simulink library "Linkage_Arms"  (R2026a)
settings: Solver=VariableStepAuto
undefined symbols (not defined in the file): Ac, Af, Ar, bcr_mass, clr_bcr, clr_conn_la, clr_conn_pullrod, clr_conn_rod, clr_la, clr_laf, clr_lar, clr_pullrod, clr_rod, clr_ua, hp_arb, hp_bcr_pivot, hp_bcr_shock_heave, hp_bcr_shock_roll, hp_in_f_la, hp_in_f_ua, hp_in_r_la, hp_in_r_ua, hp_la_arb, hp_out_f_la, hp_out_la, hp_out_r_la, hp_out_ua, hp_pullrod_in, hp_pullrod_out, hp_pushrod_in, hp_spr_bcr, hp_spr_bot, hp_uar_rod, hp_upr_rod, la_mass, laf_mass, lar_mass, opc_bcr, opc_conn_la, opc_conn_pullrod, opc_conn_rod, opc_la, opc_laf, opc_lar, opc_pullrod, opc_rod, opc_ua, pullrod_mass, radius_bcr, radius_la, radius_laf, radius_lar, radius_pullrod, radius_rod, radius_ua, rod_mass, size_conn_la, size_conn_pullrod, size_conn_rod, ua_mass ... (+3)
libraries: Suspension_Utilities x29, sm_lib x25
(part 1 of 2)
Description:
  | Component of Simscape Vehicle Templates Library
  | 
  | Copyright 2018-2026 The MathWorks, Inc.
settings Model: Creator=smiller  LastModifiedBy=smiller

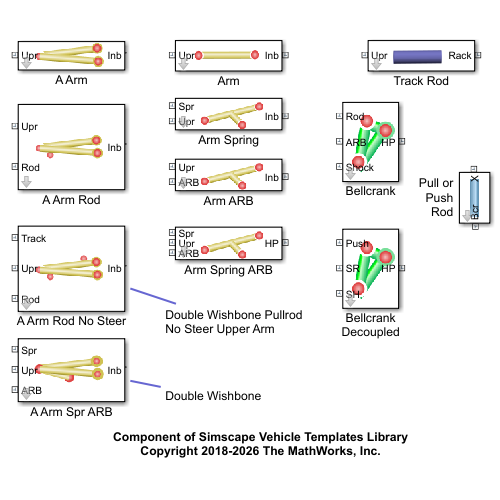
[thumbnail: Simulink's stored preview of the top-level diagram]
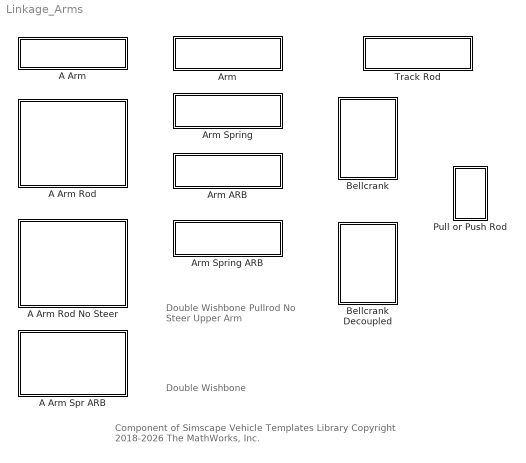
== system Linkage_Arms ==
  note: Component of Simscape Vehicle Templates Library
      | Copyright 2018-2026 The MathWorks, Inc.
  note: Double Wishbone Pullrod
      | No Steer Upper Arm
  note: Double Wishbone
  A Arm : Subsystem  mask(A-Arm){popup_leftRight=Left, hp_in_f=hp_in_f_ua, hp_in_r=hp_in_r_ua, hp_out=hp_out_ua, arm_mass=ua_mass, clr_arm=clr_ua, opc_arm=opc_ua, radius_arm=radius_ua}
      mask prompts: popup_leftRight "Left/Right"; hp_in_f "Inboard Front [xyz] (m)"; hp_in_r "Inboard Rear [xyz] (m)"; hp_out "Outboard [xyz] (m)"; arm_mass "Mass (kg)"; clr_arm "Color [RGB]"; opc_arm "Opacity (0-1)"; radius_arm "Radius (m)"
      mask help: This subsystem models a A-arm for a vehicle suspension. It can be configured to have one or two attachment points to the chassis. There are connections to the chassis and the upright.
      mask init:
      | if(popup_leftRight == 1)
      |     rhs_susp = 1;
      | elseif(popup_leftRight == 2)
      |     rhs_susp = -1;
      | end
      | 
      | rhs_hp = [1 rhs_susp 1];
      mask TypeOptions popup_leftRight: Left | Right
      mask TypeOptions clr_arm: Arm F/clr_solid | Arm R/clr_solid
      mask TypeOptions opc_arm: Arm F/opc_solid | Arm R/opc_solid
      mask TypeOptions radius_arm: Arm F/rad_solid | Arm R/rad_solid
      mask DialogControl cont_a_arm Prompt: A-Arm
      mask DialogControl cont_vis_arm Prompt: Visualization
      mask Display: image('sm_car_vehicle_linkage_dw_ua_IMAGE.png');
  A Arm Rod : Subsystem  mask(A-Arm with Rod Connection){popup_leftRight=Left, hp_in_f=hp_in_f_ua, hp_in_r=hp_in_r_ua, hp_out=hp_out_ua, hp_rod=hp_pullrod_out, arm_mass=ua_mass, clr_arm=clr_ua, opc_arm=opc_ua, radius_arm=radius_ua}
      mask prompts: popup_leftRight "Left/Right"; hp_in_f "Inboard Front [xyz] (m)"; hp_in_r "Inboard Rear [xyz] (m)"; hp_out "Outboard [xyz] (m)"; hp_rod "Rod [xyz] (m)"; arm_mass "Mass (kg)"; clr_arm "Color [RGB]"; opc_arm "Opacity (0-1)"; radius_arm "Radius (m)"
      mask help: This subsystem models a A-arm for a vehicle suspension. It can be configured to have one or two attachment points to the chassis. There are frames for connecting to the chassis, upright and a rod.
      mask init:
      | if(popup_leftRight == 1)
      |     rhs_susp = 1;
      | elseif(popup_leftRight == 2)
      |     rhs_susp = -1;
      | end
      | 
      | rhs_hp = [1 rhs_susp 1];
      mask TypeOptions popup_leftRight: Left | Right
      mask TypeOptions clr_arm: Arm F/clr_solid | Arm R/clr_solid
      mask TypeOptions opc_arm: Arm F/opc_solid | Arm R/opc_solid
      mask TypeOptions radius_arm: Arm F/rad_solid | Arm R/rad_solid
      mask DialogControl cont_a_arm Prompt: A-Arm
      mask DialogControl cont_vis_arm Prompt: Visualization
      mask Display: image('sm_car_vehicle_linkage_dw_pullrod_ua_IMAGE.png');
  A Arm Rod No Steer : Subsystem  mask(A-Arm with Rod and Track Rod Connections){popup_leftRight=Left, hp_in_f=hp_in_f_ua, hp_in_r=hp_in_r_ua, hp_r_upr=hp_uar_rod, hp_out=hp_out_ua, hp_rod=hp_pullrod_out, ua_mass=ua_mass, clr_solid=clr_ua, opc_solid=opc_ua, rad_solid=radius_ua}
      mask prompts: popup_leftRight "Left/Right"; hp_in_f "Inboard Front [xyz] (m)"; hp_in_r "Inboard Rear [xyz] (m)"; hp_r_upr "Inboard Rear to Upright [xyz] (m)"; hp_out "Outboard [xyz] (m)"; hp_rod "Rod [xyz] (m)"; ua_mass "Mass (kg)"; clr_solid "Color [RGB]"; opc_solid "Opacity (0-1)"; rad_solid "Radius (m)"
      mask help: This subsystem models a A-arm for a vehicle suspension. It can be configured to have one or two attachment points to the chassis. There are frames for connecting to the chassis, upright, rod, and track rod.
      mask init:
      | if(popup_leftRight == 1)
      |     rhs_susp = 1;
      | elseif(popup_leftRight == 2)
      |     rhs_susp = -1;
      | end
      | 
      | rhs_hp = [1 rhs_susp 1];
      mask TypeOptions popup_leftRight: Left | Right
      mask TypeOptions clr_solid: Arm F/clr_solid | Arm R/clr_solid | Arm Rod/clr_solid
      mask TypeOptions opc_solid: Arm F/opc_solid | Arm R/opc_solid | Arm Rod/opc_solid
      mask TypeOptions rad_solid: Arm F/rad_solid | Arm R/rad_solid | Arm Rod/rad_solid
      mask DialogControl cont_a_arm Prompt: A-Arm
      mask DialogControl cont_vis_ua Prompt: Visualization
      mask Display: image('sm_car_vehicle_linkage_dw_pullrod_noSteer_ua_IMAGE.png');
  A Arm Spr ARB : Subsystem  mask(A-Arm with Spring and ARB attachment){popup_leftRight=Left, hp_in_f=hp_in_f_la, hp_in_r=hp_in_r_la, hp_out=hp_out_la, hp_spr=hp_spr_bot, hp_arb=hp_la_arb, arm_mass=la_mass, clr_arm=clr_la, opc_arm=opc_la, radius_arm=radius_la}
      mask prompts: popup_leftRight "Left/Right"; hp_in_f "Inboard Front [xyz] (m)"; hp_in_r "Inboard Rear [xyz] (m)"; hp_out "Outboard [xyz] (m)"; hp_spr "Spring [xyz] (m)"; hp_arb "Anti-Roll Bar [xyz] (m)"; arm_mass "Mass (kg)"; clr_arm "Color [RGB]"; opc_arm "Opacity (0-1)"; radius_arm "Radius (m)"
      mask help: This subsystem models an arm of a wishbone suspension. It can be configured to have one or two attachment points to the chassis. There are connections to the upright, spring, and anti-roll bar.
      mask init:
      | % Set parameter for mirroring (+y or -y)
      | if(popup_leftRight == 1)
      |     rhs_susp = 1;
      | elseif(popup_leftRight == 2)
      |     rhs_susp = -1;
      | end
      | 
      | rhs_hp = [1 rhs_susp 1];
      mask Help: web ('sm_car_lower_arm_help.html')
      mask TypeOptions popup_leftRight: Left | Right
      mask TypeOptions clr_arm: Arm ARB/clr_solid | Arm F/clr_solid | Arm R/clr_solid | Arm Spring/clr_solid
      mask TypeOptions opc_arm: Arm ARB/opc_solid | Arm F/opc_solid | Arm R/opc_solid | Arm Spring/opc_solid
      mask TypeOptions radius_arm: Arm ARB/rad_solid | Arm F/rad_solid | Arm R/rad_solid | Arm Spring/rad_solid
      mask DialogControl cont_a_arm Prompt: A-Arm
      mask DialogControl cont_vis_arm Prompt: Visualization
      mask Display: image('sm_car_vehicle_linkage_dw_la_IMAGE.png');
  Arm : Subsystem  VariantControl=Steer  mask(Arm){popup_leftRight=Left, hp_in=hp_in_r_la, hp_out=hp_out_r_la, rod_mass=lar_mass, clr_conn_rod=clr_conn_la, opc_conn_rod=opc_conn_la, size_conn_rod=size_conn_la, clr_rod=clr_lar, opc_rod=opc_lar, radius_rod=radius_lar}
      mask prompts: popup_leftRight "Left/Right"; hp_in "Inboard [xyz] (m)"; hp_out "Outboard [xyz] (m)"; rod_mass "Mass (kg)"
      mask help: Rigid arm with two connection points.
      mask init:
      | if(popup_leftRight == 1)
      |     rhs_rod = 1;
      | elseif(popup_leftRight == 2)
      |     rhs_rod = -1;
      | end
      mask TypeOptions popup_leftRight: Left | Right
      mask TypeOptions rod_mass: Arm/Mass
      mask TypeOptions clr_conn_rod:
      | Vis
      | HP
      | Upr/GraphicDiffuseColor | Vis
      | HP
      | Inb/GraphicDiffuseColor
      mask TypeOptions opc_conn_rod:
      | Vis
      | HP
      | Upr/GraphicOpacity | Vis
      | HP
      | Inb/GraphicOpacity
      mask TypeOptions clr_rod: Arm/clr_solid
      mask TypeOptions opc_rod: Arm/opc_solid
      mask TypeOptions radius_rod: Arm/rad_solid
      mask DialogControl cont_rod Prompt: Rod
      mask DialogControl grp_rod Prompt: Rod
      mask DialogControl cont_vis_rod Prompt: Visualization
      mask DialogControl text_clr_rod Prompt: Color [RGB]
      mask DialogControl text_opc_rod Prompt: Opacity (0-1)
      mask DialogControl text_size_rod Prompt: Radius (m)
      mask DialogControl text_conn_rod Prompt: Connections
      mask DialogControl text_rod_rod Prompt: Rod
      mask Display: image('sm_car_vehicle_linkage_link_IMAGE.png');
  Arm ARB : Subsystem  VariantControl=Steer  mask(Arm with Anti-Roll Bar Connection){popup_leftRight=Left, hp_in=hp_in_r_la, hp_out=hp_out_r_la, hp_arb=hp_arb, rod_mass=lar_mass, clr_conn_rod=clr_conn_la, opc_conn_rod=opc_conn_la, size_conn_rod=size_conn_la, clr_rod=clr_laf, opc_rod=opc_laf, radius_rod=radius_laf}
      mask prompts: popup_leftRight "Left/Right"; hp_in "Inboard [xyz] (m)"; hp_out "Outboard [xyz] (m)"; hp_arb "ARB Mount [xyz] (m)"; rod_mass "Mass (kg)"
      mask help: Rigid arm with two ends and a frame for connecting to the anti-roll bar.
      mask init:
      | if(popup_leftRight == 1)
      |     rhs_rod = 1;
      | elseif(popup_leftRight == 2)
      |     rhs_rod = -1;
      | end
      mask TypeOptions popup_leftRight: Left | Right
      mask TypeOptions rod_mass: Arm/Mass
      mask TypeOptions clr_conn_rod:
      | Vis
      | HP
      | Upright/GraphicDiffuseColor | Vis
      | HP
      | Inb/GraphicDiffuseColor
      mask TypeOptions opc_conn_rod:
      | Vis
      | HP
      | Upright/GraphicOpacity | Vis
      | HP
      | Inb/GraphicOpacity
      mask TypeOptions clr_rod: Arm/clr_solid
      mask TypeOptions opc_rod: Arm/opc_solid
      mask TypeOptions radius_rod: Arm/rad_solid
      mask DialogControl cont_rod Prompt: Rod
      mask DialogControl grp_rod Prompt: Rod
      mask DialogControl cont_vis_rod Prompt: Visualization
      mask DialogControl text_clr_rod Prompt: Color [RGB]
      mask DialogControl text_opc_rod Prompt: Opacity (0-1)
      mask DialogControl text_size_rod Prompt: Radius (m)
      mask DialogControl text_conn_rod Prompt: Connections
      mask DialogControl text_rod_rod Prompt: Rod
      mask Display: image('sm_car_vehicle_linkage_link_s2f_IMAGE.png');
  Arm Spring : Subsystem  VariantControl=Steer  mask(Arm with Spring Connection){popup_leftRight=Left, hp_in=hp_in_f_la, hp_out=hp_out_f_la, hp_spr=hp_spr_bot, rod_mass=laf_mass, clr_conn_rod=clr_conn_la, opc_conn_rod=opc_conn_la, size_conn_rod=size_conn_la, clr_rod=clr_laf, opc_rod=opc_laf, radius_rod=radius_laf}
      mask prompts: popup_leftRight "Left/Right"; hp_in "Inboard [xyz] (m)"; hp_out "Outboard [xyz] (m)"; hp_spr "Spring Mount [xyz] (m)"; rod_mass "Mass (kg)"
      mask help: Rigid arm with two ends and a frame for connecting to the spring.
      mask init:
      | if(popup_leftRight == 1)
      |     rhs_rod = 1;
      | elseif(popup_leftRight == 2)
      |     rhs_rod = -1;
      | end
      mask TypeOptions popup_leftRight: Left | Right
      mask TypeOptions rod_mass: Arm/Mass
      mask TypeOptions clr_conn_rod:
      | Vis
      | HP
      | Upr/GraphicDiffuseColor | Vis
      | HP
      | Inb/GraphicDiffuseColor
      mask TypeOptions opc_conn_rod:
      | Vis
      | HP
      | Upr/GraphicOpacity | Vis
      | HP
      | Inb/GraphicOpacity
      mask TypeOptions clr_rod: Arm/clr_solid
      mask TypeOptions opc_rod: Arm/opc_solid
      mask TypeOptions radius_rod: Arm/rad_solid
      mask DialogControl cont_rod Prompt: Rod
      mask DialogControl grp_rod Prompt: Rod
      mask DialogControl cont_vis_rod Prompt: Visualization
      mask DialogControl text_clr_rod Prompt: Color [RGB]
      mask DialogControl text_opc_rod Prompt: Opacity (0-1)
      mask DialogControl text_size_rod Prompt: Radius (m)
      mask DialogControl text_conn_rod Prompt: Connections
      mask DialogControl text_rod_rod Prompt: Rod
      mask Display: image('sm_car_vehicle_linkage_link_s2f_IMAGE.png');
  Arm Spring ARB : Subsystem  VariantControl=Steer  mask(Arm with Connections to Spring and Anti-Roll Bar){popup_leftRight=Left, hp_in=hp_in_r_la, hp_out=hp_out_r_la, hp_spr=hp_spr_bot, hp_arb=hp_arb, rod_mass=laf_mass, clr_conn_rod=clr_conn_la, opc_conn_rod=opc_conn_la, size_conn_rod=size_conn_la, clr_rod=clr_laf, opc_rod=opc_laf, radius_rod=radius_laf}
      mask prompts: popup_leftRight "Left/Right"; hp_in "Inboard [xyz] (m)"; hp_out "Outboard [xyz] (m)"; hp_spr "Spring Mount [xyz] (m)"; hp_arb "ARB Mount [xyz] (m)"; rod_mass "Mass (kg)"
      mask help: Rigid arm with two ends and frames for connecting to the spring and anti-roll bar.
      mask init:
      | if(popup_leftRight == 1)
      |     rhs_rod = 1;
      | elseif(popup_leftRight == 2)
      |     rhs_rod = -1;
      | end
      mask TypeOptions popup_leftRight: Left | Right
      mask TypeOptions rod_mass: Arm/Mass
      mask TypeOptions clr_conn_rod:
      | Vis
      | Upright
      | Steer/GraphicDiffuseColor | Vis
      | Rack
      | Rod/GraphicDiffuseColor
      mask TypeOptions opc_conn_rod:
      | Vis
      | Upright
      | Steer/GraphicOpacity | Vis
      | Rack
      | Rod/GraphicOpacity
      mask TypeOptions clr_rod: Arm/clr_solid
      mask TypeOptions opc_rod: Arm/opc_solid
      mask TypeOptions radius_rod: Arm/rad_solid
      mask DialogControl cont_rod Prompt: Rod
      mask DialogControl grp_rod Prompt: Rod
      mask DialogControl cont_vis_rod Prompt: Visualization
      mask DialogControl text_clr_rod Prompt: Color [RGB]
      mask DialogControl text_opc_rod Prompt: Opacity (0-1)
      mask DialogControl text_size_rod Prompt: Radius (m)
      mask DialogControl text_conn_rod Prompt: Connections
      mask DialogControl text_rod_rod Prompt: Rod
      mask Display: image('sm_car_vehicle_linkage_link_s2f_IMAGE.png');
  Bellcrank : Subsystem  mask(Bellcrank){popup_leftRight=Left, hp_bcr_pivot=hp_bcr_pivot, hp_bcr_shock=hp_spr_bcr, hp_rod=hp_pullrod_in, hp_arb=hp_arb, bcr_mass=bcr_mass, clr_bcr=clr_bcr, opc_bcr=opc_bcr, radius_bcr=radius_bcr}
      mask prompts: popup_leftRight "Left/Right"; hp_bcr_pivot "HP Bellcrank Pivot [xyz] (m)"; hp_bcr_shock "HP Bellcrank Shock [xyz] (m)"; hp_rod "HP Bellcrank Rod [xyz] (m)"; hp_arb "HP Bellcrank ARB [xyz] (m)"; bcr_mass "Mass (kg)"; clr_bcr "Color [RGB]"; opc_bcr "Opacity (0-1)"; radius_bcr "Radius (m)"
      mask help: Models a bellcrank with one pivot and 3 attachment points. The axis of the pivot is normal to the plane formed by the pivot, connection to the rod, and connection to the shock.
      mask init:
      | if(popup_leftRight == 1)
      |     rhs_susp = 1;
      | elseif(popup_leftRight == 2)
      |     rhs_susp = -1;
      | end
      | 
      | rhs_hp = [1 rhs_susp 1];
      mask TypeOptions popup_leftRight: Left | Right
      mask TypeOptions clr_bcr: Arm Pivot ARB/clr_solid | Arm Pivot Rod/clr_solid | Arm Pivot Shock/clr_solid | Arm Rod Shock/clr_solid
      mask TypeOptions opc_bcr: Arm Pivot ARB/opc_solid | Arm Pivot Rod/opc_solid | Arm Pivot Shock/opc_solid | Arm Rod Shock/opc_solid
      mask TypeOptions radius_bcr: Arm Pivot ARB/rad_solid | Arm Pivot Rod/rad_solid | Arm Pivot Shock/rad_solid | Arm Rod Shock/rad_solid
      mask DialogControl cont_ua Prompt: UA
      mask DialogControl cont_vis_ua Prompt: Visualization
      mask Display: image('sm_car_vehicle_linkage_bellcrank_IMAGE.png');
  Bellcrank Decoupled : Subsystem  mask(Bellcrank){popup_leftRight=Left, hp_bcr_pivot=hp_bcr_pivot, hp_bcr_shock_heave=hp_bcr_shock_heave, hp_bcr_shock_roll=hp_bcr_shock_roll, hp_pushrod=hp_pushrod_in, bcr_mass=bcr_mass, clr_bcr=clr_bcr, opc_bcr=opc_bcr, radius_bcr=radius_bcr}
      mask prompts: popup_leftRight "Left/Right"; hp_bcr_pivot "HP Bellcrank Pivot [xyz] (m)"; hp_bcr_shock_heave "HP Bellcrank Shock Heave [xyz] (m)"; hp_bcr_shock_roll "HP Bellcrank Shock Roll [xyz] (m)"; hp_pushrod "HP Bellcrank Pushrod [xyz] (m)"; bcr_mass "Mass (kg)"; clr_bcr "Color [RGB]"; opc_bcr "Opacity (0-1)"; radius_bcr "Radius (m)"
      mask help: Models a bellcrank with one pivot and 3 attachment points. The axis of the pivot is normal to the plane formed by the pivot, connection to the pushrod, and connection to the shock.
      mask init:
      | if(popup_leftRight == 1)
      |     rhs_susp = 1;
      |     %hp_shock_roll = hp_bcr_shock_roll; % Use left value
      | elseif(popup_leftRight == 2)
      |     rhs_susp = -1;
      |     % Code to mirror hardpoint about vehicle xz plane 
      |     % and the plane defined by the bellcrank pivot axis
      |     % and the y axis of the vehicle
      |     % Code not used so that points can be specified independently
      |     % Left here as a reference.
      |     %{
      |     a1 = atan2(hp_pushrod(1)-hp_bcr_pivot(1)   ,hp_pushrod(3)-hp_bcr_pivot(3));
      |     a2 = atan2(hp_bcr_shock_roll(1)-hp_bcr_pivot(1),hp_bcr_shock_roll(3)-hp_bcr_pivot(3));
      |     d_roll2piv = norm(hp_bcr_shock_roll([1 3])-hp_bcr_pivot([1 3]));
      |     d_roll_mirror_axis = d_roll2piv*cos(a2-a1);
      |     mirr_dx = d_roll_mirror_axis*sin(a1);
      |     mirr_dz = d_roll_mirror_axis*cos(a1);
      |     hp_shock_roll = ...
      |         [hp_bcr_shock_roll(1)-2*mirr_dx -hp_bcr_shock_roll(2) hp_bcr_shock_roll(3)-2*mirr_dz];
      |     %}
      | end
      | 
      | rhs_hp = [1 rhs_susp 1];
      mask TypeOptions popup_leftRight: Left | Right
      mask TypeOptions clr_bcr: Arm Pivot Shock Roll/clr_solid | Arm Pivot Push/clr_solid | Arm Pivot Shock Heave/clr_solid | Arm Push Shock/clr_solid
      mask TypeOptions opc_bcr: Arm Pivot Shock Roll/opc_solid | Arm Pivot Push/opc_solid | Arm Pivot Shock Heave/opc_solid | Arm Push Shock/opc_solid
      mask TypeOptions radius_bcr: Arm Pivot Shock Roll/rad_solid | Arm Pivot Push/rad_solid | Arm Pivot Shock Heave/rad_solid | Arm Push Shock/rad_solid
      mask DialogControl cont_ua Prompt: UA
      mask DialogControl cont_vis_ua Prompt: Visualization
      mask Display: image('sm_car_vehicle_linkage_bellcrank_IMAGE.png');
  Pull or Push Rod : Subsystem  VariantControl=Steer  mask(Rod){popup_leftRight=Left, hp_in=hp_pullrod_in, hp_out=hp_pullrod_out, rod_mass=pullrod_mass, clr_conn_rod=clr_conn_pullrod, opc_conn_rod=opc_conn_pullrod, size_conn_rod=size_conn_pullrod, clr_rod=clr_pullrod, opc_rod=opc_pullrod, radius_rod=radius_pullrod}
      mask prompts: popup_leftRight "Left/Right"; hp_in "Bellcrank [xyz] (m)"; hp_out "Arm / Upright [xyz] (m)"; rod_mass "Mass (kg)"
      mask help: Rod connecting two hard points
      mask init:
      | if(popup_leftRight == 1)
      |     rhs_rod = 1;
      | elseif(popup_leftRight == 2)
      |     rhs_rod = -1;
      | end
      mask TypeOptions popup_leftRight: Left | Right
      mask TypeOptions rod_mass: Rod/Mass
      mask TypeOptions clr_conn_rod:
      | Vis
      | Pushrod
      | X/GraphicDiffuseColor | Vis
      | Pushrod
      | Crank/GraphicDiffuseColor
      mask TypeOptions opc_conn_rod:
      | Vis
      | Pushrod
      | X/GraphicOpacity | Vis
      | Pushrod
      | Crank/GraphicOpacity
      mask TypeOptions clr_rod: Rod/clr_solid
      mask TypeOptions opc_rod: Rod/opc_solid
      mask TypeOptions radius_rod: Rod/rad_solid
      mask DialogControl cont_rod Prompt: Rod
      mask DialogControl grp_rod Prompt: Rod
      mask DialogControl cont_vis_rod Prompt: Visualization
      mask DialogControl text_clr_rod Prompt: Color [RGB]
      mask DialogControl text_opc_rod Prompt: Opac. (0-1)
      mask DialogControl text_size_rod Prompt: Size (m)
      mask DialogControl text_conn_rod Prompt: Connections
      mask DialogControl text_rod_rod Prompt: Rod
      mask Display: image('sm_car_vehicle_linkage_pushrod_IMAGE.png');
  Track Rod : Subsystem  VariantControl=Steer  mask(Rod){popup_leftRight=Left, hp_in=hp_uar_rod, hp_out=hp_upr_rod, rod_mass=rod_mass, clr_conn_rod=clr_conn_rod, opc_conn_rod=opc_conn_rod, size_conn_rod=size_conn_rod, clr_rod=clr_rod, opc_rod=opc_rod, radius_rod=radius_rod}
      mask prompts: popup_leftRight "Left/Right"; hp_in "Inboard [xyz] (m)"; hp_out "Outboard [xyz] (m)"; rod_mass "Mass (kg)"
      mask help: Rod connecting two hard points
      mask init:
      | if(popup_leftRight == 1)
      |     rhs_rod = 1;
      | elseif(popup_leftRight == 2)
      |     rhs_rod = -1;
      | end
      mask TypeOptions popup_leftRight: Left | Right
      mask TypeOptions rod_mass: Rod/Mass
      mask TypeOptions clr_conn_rod:
      | Vis
      | Upright
      | Steer/GraphicDiffuseColor | Vis
      | Rack
      | Rod/GraphicDiffuseColor
      mask TypeOptions opc_conn_rod:
      | Vis
      | Upright
      | Steer/GraphicOpacity | Vis
      | Rack
      | Rod/GraphicOpacity
      mask TypeOptions clr_rod: Rod/clr_solid
      mask TypeOptions opc_rod: Rod/opc_solid
      mask TypeOptions radius_rod: Rod/rad_solid
      mask DialogControl cont_rod Prompt: Rod
      mask DialogControl grp_rod Prompt: Rod
      mask DialogControl cont_vis_rod Prompt: Visualization
      mask DialogControl text_clr_rod Prompt: Color [RGB]
      mask DialogControl text_opc_rod Prompt: Opac. (0-1)
      mask DialogControl text_size_rod Prompt: Size (m)
      mask DialogControl text_conn_rod Prompt: Connections
      mask DialogControl text_rod_rod Prompt: Rod
      mask Display: image('sm_car_linkage_trackrod_IMAGE.png');

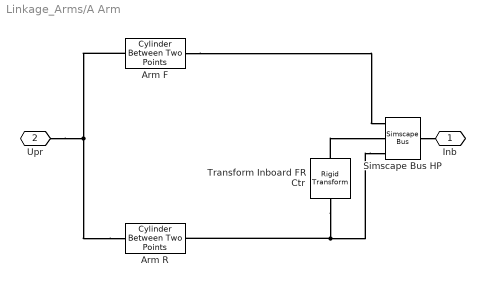
== system Linkage_Arms/A Arm ==
  Arm F : Suspension_Utilities/Cylinder Between Two Points  hp_b=hp_in_f.*rhs_hp  hp_f=hp_out.*rhs_hp  Mass=arm_mass/2  clr_solid=clr_arm  opc_solid=opc_arm  rad_solid=radius_arm
  Arm R : Suspension_Utilities/Cylinder Between Two Points  hp_b=hp_in_r.*rhs_hp  hp_f=hp_out.*rhs_hp  Mass=arm_mass/2  clr_solid=clr_arm  opc_solid=opc_arm  rad_solid=radius_arm
  Simscape Bus HP : SimscapeBus  HierarchyStrings=Af;Ac;Ar
  Transform Inboard FR Ctr : sm_lib/Frames and Transforms/Rigid Transform  RotationMethod=None  FollAlignAxisA=+X  BaseAlignAxisA=+Y  FollAlignAxisB=+Y  BaseAlignAxisB=+Z  RotationStandardAxis=+Z  RotationAngle=0.0  RotationAngleUnits=deg  RotationArbitraryAxis=[0 0 1]  RotationSequenceAxes=FollowerAxes  RotationSequence=XYX  RotationSequenceAngles=[0 0 0]  RotationSequenceAnglesUnits=deg  RotationMatrix=[1 0 0; 0 1 0; 0 0 1]  Quaternion=[1 0 0 0]  TranslationMethod=Cartesian  TranslationCartesianOffset=(hp_in_f - hp_in_r).*rhs_hp/2  TranslationCartesianOffsetUnits=m  TranslationStandardAxis=+Z  TranslationStandardOffset=0  TranslationStandardOffsetUnits=m  TranslationROffset=0  TranslationROffsetUnits=m  TranslationThetaOffset=0  TranslationThetaOffsetUnits=deg  TranslationZOffset=0  TranslationZOffsetUnits=m
  Inb : PMIOPort  Side=Right
  Upr : PMIOPort  Port=2  Side=Left
  connections:
  Arm R/RConn1 -- Upr/RConn1 -- Arm F/RConn1
  Simscape Bus HP/LConn3 -- Arm R/LConn1 -- Transform Inboard FR Ctr/LConn1
  Arm F/LConn1 -- Simscape Bus HP/LConn1
  Transform Inboard FR Ctr/RConn1 -- Simscape Bus HP/LConn2
  Simscape Bus HP/RConn1 -- Inb/RConn1

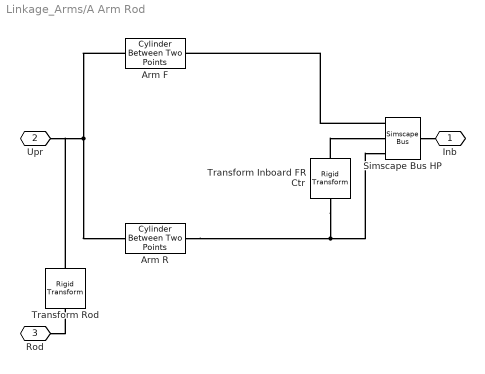
== system Linkage_Arms/A Arm Rod ==
  Arm F : Suspension_Utilities/Cylinder Between Two Points  hp_b=hp_in_f.*rhs_hp  hp_f=hp_out.*rhs_hp  Mass=ua_mass/2  clr_solid=clr_arm  opc_solid=opc_arm  rad_solid=radius_arm
  Arm R : Suspension_Utilities/Cylinder Between Two Points  hp_b=hp_in_r.*rhs_hp  hp_f=hp_out.*rhs_hp  Mass=ua_mass/2  clr_solid=clr_arm  opc_solid=opc_arm  rad_solid=radius_arm
  Simscape Bus HP : SimscapeBus  HierarchyStrings=Af;Ac;Ar
  Transform Inboard FR Ctr : sm_lib/Frames and Transforms/Rigid Transform  RotationMethod=None  FollAlignAxisA=+X  BaseAlignAxisA=+Y  FollAlignAxisB=+Y  BaseAlignAxisB=+Z  RotationStandardAxis=+Z  RotationAngle=0.0  RotationAngleUnits=deg  RotationArbitraryAxis=[0 0 1]  RotationSequenceAxes=FollowerAxes  RotationSequence=XYX  RotationSequenceAngles=[0 0 0]  RotationSequenceAnglesUnits=deg  RotationMatrix=[1 0 0; 0 1 0; 0 0 1]  Quaternion=[1 0 0 0]  TranslationMethod=Cartesian  TranslationCartesianOffset=(hp_in_f - hp_in_r).*rhs_hp/2  TranslationCartesianOffsetUnits=m  TranslationStandardAxis=+Z  TranslationStandardOffset=0  TranslationStandardOffsetUnits=m  TranslationROffset=0  TranslationROffsetUnits=m  TranslationThetaOffset=0  TranslationThetaOffsetUnits=deg  TranslationZOffset=0  TranslationZOffsetUnits=m
  Transform Rod : sm_lib/Frames and Transforms/Rigid Transform  RotationMethod=None  FollAlignAxisA=+X  BaseAlignAxisA=+Y  FollAlignAxisB=+Y  BaseAlignAxisB=+Z  RotationStandardAxis=+Z  RotationAngle=0.0  RotationAngleUnits=deg  RotationArbitraryAxis=[0 0 1]  RotationSequenceAxes=FollowerAxes  RotationSequence=XYX  RotationSequenceAngles=[0 0 0]  RotationSequenceAnglesUnits=deg  RotationMatrix=[1 0 0; 0 1 0; 0 0 1]  Quaternion=[1 0 0 0]  TranslationMethod=Cartesian  TranslationCartesianOffset=(hp_rod-hp_out).*rhs_hp  TranslationCartesianOffsetUnits=m  TranslationStandardAxis=+Z  TranslationStandardOffset=0  TranslationStandardOffsetUnits=m  TranslationROffset=0  TranslationROffsetUnits=m  TranslationThetaOffset=0  TranslationThetaOffsetUnits=deg  TranslationZOffset=0  TranslationZOffsetUnits=m
  Inb : PMIOPort  Side=Right
  Upr : PMIOPort  Port=2  Side=Left
  Rod : PMIOPort  Port=3  Side=Left
  connections:
  Rod/RConn1 -- Transform Rod/RConn1
  Simscape Bus HP/RConn1 -- Inb/RConn1
  Transform Inboard FR Ctr/RConn1 -- Simscape Bus HP/LConn2
  Transform Inboard FR Ctr/LConn1 -- Simscape Bus HP/LConn3 -- Arm R/LConn1
  Simscape Bus HP/LConn1 -- Arm F/LConn1
  Arm F/RConn1 -- Upr/RConn1 -- Transform Rod/LConn1 -- Arm R/RConn1

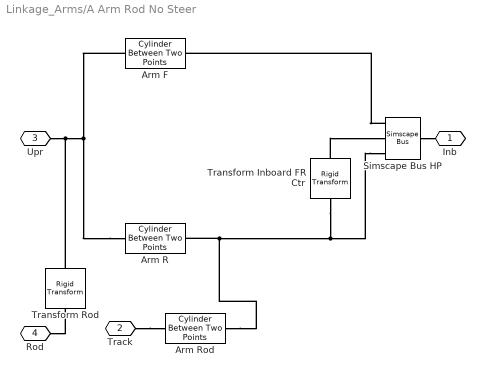
== system Linkage_Arms/A Arm Rod No Steer ==
  Arm F : Suspension_Utilities/Cylinder Between Two Points  hp_b=hp_in_f.*rhs_hp  hp_f=hp_out.*rhs_hp  Mass=ua_mass/2  clr_solid=clr_solid  opc_solid=opc_solid  rad_solid=rad_solid
  Arm R : Suspension_Utilities/Cylinder Between Two Points  hp_b=hp_in_r.*rhs_hp  hp_f=hp_out.*rhs_hp  Mass=ua_mass/2  clr_solid=clr_solid  opc_solid=opc_solid  rad_solid=rad_solid
  Arm Rod : Suspension_Utilities/Cylinder Between Two Points  hp_b=hp_in_r.*rhs_hp  hp_f=hp_r_upr.*rhs_hp  Mass=0  clr_solid=clr_solid  opc_solid=opc_solid  rad_solid=rad_solid
  Simscape Bus HP : SimscapeBus  HierarchyStrings=Af;Ac;Ar
  Transform Inboard FR Ctr : sm_lib/Frames and Transforms/Rigid Transform  RotationMethod=None  FollAlignAxisA=+X  BaseAlignAxisA=+Y  FollAlignAxisB=+Y  BaseAlignAxisB=+Z  RotationStandardAxis=+Z  RotationAngle=0.0  RotationAngleUnits=deg  RotationArbitraryAxis=[0 0 1]  RotationSequenceAxes=FollowerAxes  RotationSequence=XYX  RotationSequenceAngles=[0 0 0]  RotationSequenceAnglesUnits=deg  RotationMatrix=[1 0 0; 0 1 0; 0 0 1]  Quaternion=[1 0 0 0]  TranslationMethod=Cartesian  TranslationCartesianOffset=(hp_in_f - hp_in_r).*rhs_hp/2  TranslationCartesianOffsetUnits=m  TranslationStandardAxis=+Z  TranslationStandardOffset=0  TranslationStandardOffsetUnits=m  TranslationROffset=0  TranslationROffsetUnits=m  TranslationThetaOffset=0  TranslationThetaOffsetUnits=deg  TranslationZOffset=0  TranslationZOffsetUnits=m
  Transform Rod : sm_lib/Frames and Transforms/Rigid Transform  RotationMethod=None  FollAlignAxisA=+X  BaseAlignAxisA=+Y  FollAlignAxisB=+Y  BaseAlignAxisB=+Z  RotationStandardAxis=+Z  RotationAngle=0.0  RotationAngleUnits=deg  RotationArbitraryAxis=[0 0 1]  RotationSequenceAxes=FollowerAxes  RotationSequence=XYX  RotationSequenceAngles=[0 0 0]  RotationSequenceAnglesUnits=deg  RotationMatrix=[1 0 0; 0 1 0; 0 0 1]  Quaternion=[1 0 0 0]  TranslationMethod=Cartesian  TranslationCartesianOffset=(hp_rod-hp_out).*rhs_hp  TranslationCartesianOffsetUnits=m  TranslationStandardAxis=+Z  TranslationStandardOffset=0  TranslationStandardOffsetUnits=m  TranslationROffset=0  TranslationROffsetUnits=m  TranslationThetaOffset=0  TranslationThetaOffsetUnits=deg  TranslationZOffset=0  TranslationZOffsetUnits=m
  Inb : PMIOPort  Side=Right
  Track : PMIOPort  Port=2  Side=Left
  Upr : PMIOPort  Port=3  Side=Left
  Rod : PMIOPort  Port=4  Side=Left
  connections:
  Track/RConn1 -- Arm Rod/RConn1
  Arm R/RConn1 -- Transform Rod/LConn1 -- Upr/RConn1 -- Arm F/RConn1
  Simscape Bus HP/LConn1 -- Arm F/LConn1
  Simscape Bus HP/LConn3 -- Transform Inboard FR Ctr/LConn1 -- Arm R/LConn1 -- Arm Rod/LConn1
  Transform Inboard FR Ctr/RConn1 -- Simscape Bus HP/LConn2
  Simscape Bus HP/RConn1 -- Inb/RConn1
  Rod/RConn1 -- Transform Rod/RConn1

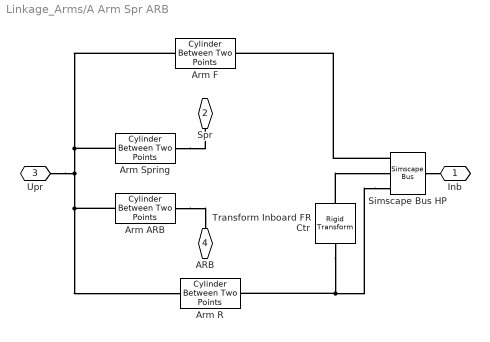
== system Linkage_Arms/A Arm Spr ARB ==
  Arm ARB : Suspension_Utilities/Cylinder Between Two Points  hp_b=hp_arb.*rhs_hp  hp_f=hp_out.*rhs_hp  Mass=0  clr_solid=clr_arm  opc_solid=opc_arm  rad_solid=radius_arm
  Arm F : Suspension_Utilities/Cylinder Between Two Points  hp_b=hp_in_f.*rhs_hp  hp_f=hp_out.*rhs_hp  Mass=arm_mass/2  clr_solid=clr_arm  opc_solid=opc_arm  rad_solid=radius_arm
  Arm R : Suspension_Utilities/Cylinder Between Two Points  hp_b=hp_in_r.*rhs_hp  hp_f=hp_out.*rhs_hp  Mass=arm_mass/2  clr_solid=clr_arm  opc_solid=opc_arm  rad_solid=radius_arm
  Arm Spring : Suspension_Utilities/Cylinder Between Two Points  hp_b=hp_spr.*rhs_hp  hp_f=hp_out.*rhs_hp  Mass=0  clr_solid=clr_arm  opc_solid=opc_arm  rad_solid=radius_arm
  Simscape Bus HP : SimscapeBus  HierarchyStrings=Af;Ac;Ar
  Transform Inboard FR Ctr : sm_lib/Frames and Transforms/Rigid Transform  RotationMethod=None  FollAlignAxisA=+X  BaseAlignAxisA=+Y  FollAlignAxisB=+Y  BaseAlignAxisB=+Z  RotationStandardAxis=+Z  RotationAngle=0.0  RotationAngleUnits=deg  RotationArbitraryAxis=[0 0 1]  RotationSequenceAxes=FollowerAxes  RotationSequence=XYX  RotationSequenceAngles=[0 0 0]  RotationSequenceAnglesUnits=deg  RotationMatrix=[1 0 0; 0 1 0; 0 0 1]  Quaternion=[1 0 0 0]  TranslationMethod=Cartesian  TranslationCartesianOffset=(hp_in_f - hp_in_r).*rhs_hp/2  TranslationCartesianOffsetUnits=m  TranslationStandardAxis=+Z  TranslationStandardOffset=0  TranslationStandardOffsetUnits=m  TranslationROffset=0  TranslationROffsetUnits=m  TranslationThetaOffset=0  TranslationThetaOffsetUnits=deg  TranslationZOffset=0  TranslationZOffsetUnits=m
  Inb : PMIOPort  Side=Right
  Spr : PMIOPort  Port=2  Side=Left
  Upr : PMIOPort  Port=3  Side=Left
  ARB : PMIOPort  Port=4  Side=Left
  connections:
  Transform Inboard FR Ctr/RConn1 -- Simscape Bus HP/LConn2
  Simscape Bus HP/RConn1 -- Inb/RConn1
  Arm Spring/LConn1 -- Spr/RConn1
  Arm F/RConn1 -- Arm R/RConn1 -- Arm ARB/RConn1 -- Upr/RConn1 -- Arm Spring/RConn1
  Simscape Bus HP/LConn3 -- Transform Inboard FR Ctr/LConn1 -- Arm R/LConn1
  Simscape Bus HP/LConn1 -- Arm F/LConn1
  Arm ARB/LConn1 -- ARB/RConn1

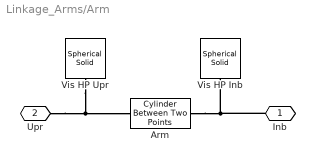
== system Linkage_Arms/Arm ==
  Arm : Suspension_Utilities/Cylinder Between Two Points  hp_b=hp_in.*[1 rhs_rod 1]  hp_f=hp_out.*[1 rhs_rod 1]  Mass=rod_mass  clr_solid=clr_rod  opc_solid=opc_rod  rad_solid=radius_rod
  Vis HP Inb : sm_lib/Body Elements/Spherical Solid  SphereRadius=size_conn_rod  SphereRadiusUnits=m  ExportEntireGeometry=off  InertiaType=CalculateFromGeometry  BasedOnType=Density  Density=0  DensityUnits=kg/m^3  Mass=1  MassUnits=kg  CenterOfMass=[0 0 0]  CenterOfMassUnits=m  MomentsOfInertia=[1 1 1]  MomentsOfInertiaUnits=kg*m^2  ProductsOfInertia=[0 0 0]  ProductsOfInertiaUnits=kg*m^2  GraphicType=FromGeometry  MarkerShape=Sphere  MarkerSize=10  GraphicVisPropType=SimpleVisualProperties  GraphicDiffuseColor=clr_conn_rod  GraphicOpacity=opc_conn_rod  GraphicSpecularColor=[0.5 0.5 0.5 1.0]  GraphicAmbientColor=[0.15 0.15 0.15 1.0]  GraphicEmissiveColor=[0.0 0.0 0.0 1.0]  GraphicShininess=75  DoExposeReferenceFrame=on  SerializedFrames=<Frames/>
  Vis HP Upr : sm_lib/Body Elements/Spherical Solid  SphereRadius=size_conn_rod  SphereRadiusUnits=m  ExportEntireGeometry=off  InertiaType=CalculateFromGeometry  BasedOnType=Density  Density=0  DensityUnits=kg/m^3  Mass=1  MassUnits=kg  CenterOfMass=[0 0 0]  CenterOfMassUnits=m  MomentsOfInertia=[1 1 1]  MomentsOfInertiaUnits=kg*m^2  ProductsOfInertia=[0 0 0]  ProductsOfInertiaUnits=kg*m^2  GraphicType=FromGeometry  MarkerShape=Sphere  MarkerSize=10  GraphicVisPropType=SimpleVisualProperties  GraphicDiffuseColor=clr_conn_rod  GraphicOpacity=opc_conn_rod  GraphicSpecularColor=[0.5 0.5 0.5 1.0]  GraphicAmbientColor=[0.15 0.15 0.15 1.0]  GraphicEmissiveColor=[0.0 0.0 0.0 1.0]  GraphicShininess=75  DoExposeReferenceFrame=on  SerializedFrames=<Frames/>
  Inb : PMIOPort  Side=Right
  Upr : PMIOPort  Port=2  Side=Left
  connections:
  Arm/LConn1 -- Inb/RConn1 -- Vis HP Inb/RConn1
  Upr/RConn1 -- Arm/RConn1 -- Vis HP Upr/RConn1

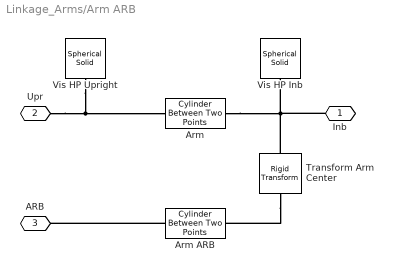
== system Linkage_Arms/Arm ARB ==
  Arm : Suspension_Utilities/Cylinder Between Two Points  hp_b=hp_in.*[1 rhs_rod 1]  hp_f=hp_out.*[1 rhs_rod 1]  Mass=rod_mass  clr_solid=clr_rod  opc_solid=opc_rod  rad_solid=radius_rod
  Arm ARB : Suspension_Utilities/Cylinder Between Two Points  hp_b=0.5*(hp_in+hp_out).*[1, rhs_rod, 1]  hp_f=hp_arb.*[1, rhs_rod, 1]  Mass=1e-5  clr_solid=clr_rod  opc_solid=opc_rod  rad_solid=radius_rod
  Transform Arm Center : sm_lib/Frames and Transforms/Rigid Transform  RotationMethod=None  FollAlignAxisA=+X  BaseAlignAxisA=+Y  FollAlignAxisB=+Y  BaseAlignAxisB=+Z  RotationStandardAxis=+Z  RotationAngle=0.0  RotationAngleUnits=deg  RotationArbitraryAxis=[0 0 1]  RotationSequenceAxes=FollowerAxes  RotationSequence=XYX  RotationSequenceAngles=[0 0 0]  RotationSequenceAnglesUnits=deg  RotationMatrix=[1 0 0; 0 1 0; 0 0 1]  Quaternion=[1 0 0 0]  TranslationMethod=Cartesian  TranslationCartesianOffset=0.5*(hp_out-hp_in).*[1, rhs_rod, 1]  TranslationCartesianOffsetUnits=m  TranslationStandardAxis=+Z  TranslationStandardOffset=0  TranslationStandardOffsetUnits=m  TranslationROffset=0  TranslationROffsetUnits=m  TranslationThetaOffset=0  TranslationThetaOffsetUnits=deg  TranslationZOffset=0  TranslationZOffsetUnits=m
  Vis HP Inb : sm_lib/Body Elements/Spherical Solid  SphereRadius=size_conn_rod  SphereRadiusUnits=m  ExportEntireGeometry=off  InertiaType=CalculateFromGeometry  BasedOnType=Density  Density=0  DensityUnits=kg/m^3  Mass=1  MassUnits=kg  CenterOfMass=[0 0 0]  CenterOfMassUnits=m  MomentsOfInertia=[1 1 1]  MomentsOfInertiaUnits=kg*m^2  ProductsOfInertia=[0 0 0]  ProductsOfInertiaUnits=kg*m^2  GraphicType=FromGeometry  MarkerShape=Sphere  MarkerSize=10  GraphicVisPropType=SimpleVisualProperties  GraphicDiffuseColor=clr_conn_rod  GraphicOpacity=opc_conn_rod  GraphicSpecularColor=[0.5 0.5 0.5 1.0]  GraphicAmbientColor=[0.15 0.15 0.15 1.0]  GraphicEmissiveColor=[0.0 0.0 0.0 1.0]  GraphicShininess=75  DoExposeReferenceFrame=on  SerializedFrames=<Frames/>
  Vis HP Upright : sm_lib/Body Elements/Spherical Solid  SphereRadius=size_conn_rod  SphereRadiusUnits=m  ExportEntireGeometry=off  InertiaType=CalculateFromGeometry  BasedOnType=Density  Density=0  DensityUnits=kg/m^3  Mass=1  MassUnits=kg  CenterOfMass=[0 0 0]  CenterOfMassUnits=m  MomentsOfInertia=[1 1 1]  MomentsOfInertiaUnits=kg*m^2  ProductsOfInertia=[0 0 0]  ProductsOfInertiaUnits=kg*m^2  GraphicType=FromGeometry  MarkerShape=Sphere  MarkerSize=10  GraphicVisPropType=SimpleVisualProperties  GraphicDiffuseColor=clr_conn_rod  GraphicOpacity=opc_conn_rod  GraphicSpecularColor=[0.5 0.5 0.5 1.0]  GraphicAmbientColor=[0.15 0.15 0.15 1.0]  GraphicEmissiveColor=[0.0 0.0 0.0 1.0]  GraphicShininess=75  DoExposeReferenceFrame=on  SerializedFrames=<Frames/>
  Inb : PMIOPort  Side=Right
  Upr : PMIOPort  Port=2  Side=Left
  ARB : PMIOPort  Port=3  Side=Left
  connections:
  Transform Arm Center/RConn1 -- Arm ARB/LConn1
  Arm ARB/RConn1 -- ARB/RConn1
  Vis HP Upright/RConn1 -- Arm/RConn1 -- Upr/RConn1
  Transform Arm Center/LConn1 -- Inb/RConn1 -- Arm/LConn1 -- Vis HP Inb/RConn1

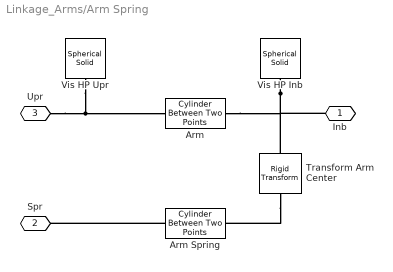
== system Linkage_Arms/Arm Spring ==
  Arm : Suspension_Utilities/Cylinder Between Two Points  hp_b=hp_in.*[1 rhs_rod 1]  hp_f=hp_out.*[1 rhs_rod 1]  Mass=rod_mass  clr_solid=clr_rod  opc_solid=opc_rod  rad_solid=radius_rod
  Arm Spring : Suspension_Utilities/Cylinder Between Two Points  hp_b=0.5*(hp_in+hp_out).*[1, rhs_rod, 1]  hp_f=hp_spr.*[1, rhs_rod, 1]  Mass=1e-5  clr_solid=clr_rod  opc_solid=opc_rod  rad_solid=radius_rod
  Transform Arm Center : sm_lib/Frames and Transforms/Rigid Transform  RotationMethod=None  FollAlignAxisA=+X  BaseAlignAxisA=+Y  FollAlignAxisB=+Y  BaseAlignAxisB=+Z  RotationStandardAxis=+Z  RotationAngle=0.0  RotationAngleUnits=deg  RotationArbitraryAxis=[0 0 1]  RotationSequenceAxes=FollowerAxes  RotationSequence=XYX  RotationSequenceAngles=[0 0 0]  RotationSequenceAnglesUnits=deg  RotationMatrix=[1 0 0; 0 1 0; 0 0 1]  Quaternion=[1 0 0 0]  TranslationMethod=Cartesian  TranslationCartesianOffset=0.5*(hp_out-hp_in).*[1, rhs_rod, 1]  TranslationCartesianOffsetUnits=m  TranslationStandardAxis=+Z  TranslationStandardOffset=0  TranslationStandardOffsetUnits=m  TranslationROffset=0  TranslationROffsetUnits=m  TranslationThetaOffset=0  TranslationThetaOffsetUnits=deg  TranslationZOffset=0  TranslationZOffsetUnits=m
  Vis HP Inb : sm_lib/Body Elements/Spherical Solid  SphereRadius=size_conn_rod  SphereRadiusUnits=m  ExportEntireGeometry=off  InertiaType=CalculateFromGeometry  BasedOnType=Density  Density=0  DensityUnits=kg/m^3  Mass=1  MassUnits=kg  CenterOfMass=[0 0 0]  CenterOfMassUnits=m  MomentsOfInertia=[1 1 1]  MomentsOfInertiaUnits=kg*m^2  ProductsOfInertia=[0 0 0]  ProductsOfInertiaUnits=kg*m^2  GraphicType=FromGeometry  MarkerShape=Sphere  MarkerSize=10  GraphicVisPropType=SimpleVisualProperties  GraphicDiffuseColor=clr_conn_rod  GraphicOpacity=opc_conn_rod  GraphicSpecularColor=[0.5 0.5 0.5 1.0]  GraphicAmbientColor=[0.15 0.15 0.15 1.0]  GraphicEmissiveColor=[0.0 0.0 0.0 1.0]  GraphicShininess=75  DoExposeReferenceFrame=on  SerializedFrames=<Frames/>
  Vis HP Upr : sm_lib/Body Elements/Spherical Solid  SphereRadius=size_conn_rod  SphereRadiusUnits=m  ExportEntireGeometry=off  InertiaType=CalculateFromGeometry  BasedOnType=Density  Density=0  DensityUnits=kg/m^3  Mass=1  MassUnits=kg  CenterOfMass=[0 0 0]  CenterOfMassUnits=m  MomentsOfInertia=[1 1 1]  MomentsOfInertiaUnits=kg*m^2  ProductsOfInertia=[0 0 0]  ProductsOfInertiaUnits=kg*m^2  GraphicType=FromGeometry  MarkerShape=Sphere  MarkerSize=10  GraphicVisPropType=SimpleVisualProperties  GraphicDiffuseColor=clr_conn_rod  GraphicOpacity=opc_conn_rod  GraphicSpecularColor=[0.5 0.5 0.5 1.0]  GraphicAmbientColor=[0.15 0.15 0.15 1.0]  GraphicEmissiveColor=[0.0 0.0 0.0 1.0]  GraphicShininess=75  DoExposeReferenceFrame=on  SerializedFrames=<Frames/>
  Inb : PMIOPort  Side=Right
  Spr : PMIOPort  Port=2  Side=Left
  Upr : PMIOPort  Port=3  Side=Left
  connections:
  Vis HP Inb/RConn1 -- Arm/LConn1 -- Inb/RConn1 -- Transform Arm Center/LConn1
  Upr/RConn1 -- Arm/RConn1 -- Vis HP Upr/RConn1
  Arm Spring/RConn1 -- Spr/RConn1
  Transform Arm Center/RConn1 -- Arm Spring/LConn1

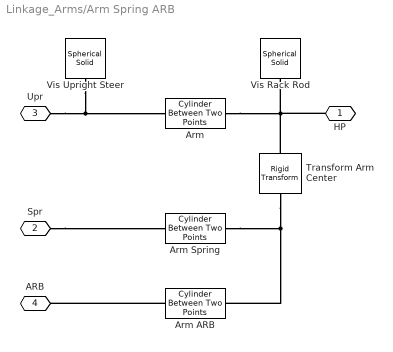
== system Linkage_Arms/Arm Spring ARB ==
  Arm : Suspension_Utilities/Cylinder Between Two Points  hp_b=hp_in.*[1 rhs_rod 1]  hp_f=hp_out.*[1 rhs_rod 1]  Mass=rod_mass  clr_solid=clr_rod  opc_solid=opc_rod  rad_solid=radius_rod
  Arm ARB : Suspension_Utilities/Cylinder Between Two Points  hp_b=0.5*(hp_in+hp_out).*[1, rhs_rod, 1]  hp_f=hp_arb.*[1, rhs_rod, 1]  Mass=1e-5  clr_solid=clr_rod  opc_solid=opc_rod  rad_solid=radius_rod
  Arm Spring : Suspension_Utilities/Cylinder Between Two Points  hp_b=0.5*(hp_in+hp_out).*[1, rhs_rod, 1]  hp_f=hp_spr.*[1, rhs_rod, 1]  Mass=1e-5  clr_solid=clr_rod  opc_solid=opc_rod  rad_solid=radius_rod
  Transform Arm Center : sm_lib/Frames and Transforms/Rigid Transform  RotationMethod=None  FollAlignAxisA=+X  BaseAlignAxisA=+Y  FollAlignAxisB=+Y  BaseAlignAxisB=+Z  RotationStandardAxis=+Z  RotationAngle=0.0  RotationAngleUnits=deg  RotationArbitraryAxis=[0 0 1]  RotationSequenceAxes=FollowerAxes  RotationSequence=XYX  RotationSequenceAngles=[0 0 0]  RotationSequenceAnglesUnits=deg  RotationMatrix=[1 0 0; 0 1 0; 0 0 1]  Quaternion=[1 0 0 0]  TranslationMethod=Cartesian  TranslationCartesianOffset=0.5*(hp_out-hp_in).*[1, rhs_rod, 1]  TranslationCartesianOffsetUnits=m  TranslationStandardAxis=+Z  TranslationStandardOffset=0  TranslationStandardOffsetUnits=m  TranslationROffset=0  TranslationROffsetUnits=m  TranslationThetaOffset=0  TranslationThetaOffsetUnits=deg  TranslationZOffset=0  TranslationZOffsetUnits=m
  Vis Rack Rod : sm_lib/Body Elements/Spherical Solid  SphereRadius=size_conn_rod  SphereRadiusUnits=m  ExportEntireGeometry=off  InertiaType=CalculateFromGeometry  BasedOnType=Density  Density=0  DensityUnits=kg/m^3  Mass=1  MassUnits=kg  CenterOfMass=[0 0 0]  CenterOfMassUnits=m  MomentsOfInertia=[1 1 1]  MomentsOfInertiaUnits=kg*m^2  ProductsOfInertia=[0 0 0]  ProductsOfInertiaUnits=kg*m^2  GraphicType=FromGeometry  MarkerShape=Sphere  MarkerSize=10  GraphicVisPropType=SimpleVisualProperties  GraphicDiffuseColor=clr_conn_rod  GraphicOpacity=opc_conn_rod  GraphicSpecularColor=[0.5 0.5 0.5 1.0]  GraphicAmbientColor=[0.15 0.15 0.15 1.0]  GraphicEmissiveColor=[0.0 0.0 0.0 1.0]  GraphicShininess=75  DoExposeReferenceFrame=on  SerializedFrames=<Frames/>
  Vis Upright Steer : sm_lib/Body Elements/Spherical Solid  SphereRadius=size_conn_rod  SphereRadiusUnits=m  ExportEntireGeometry=off  InertiaType=CalculateFromGeometry  BasedOnType=Density  Density=0  DensityUnits=kg/m^3  Mass=1  MassUnits=kg  CenterOfMass=[0 0 0]  CenterOfMassUnits=m  MomentsOfInertia=[1 1 1]  MomentsOfInertiaUnits=kg*m^2  ProductsOfInertia=[0 0 0]  ProductsOfInertiaUnits=kg*m^2  GraphicType=FromGeometry  MarkerShape=Sphere  MarkerSize=10  GraphicVisPropType=SimpleVisualProperties  GraphicDiffuseColor=clr_conn_rod  GraphicOpacity=opc_conn_rod  GraphicSpecularColor=[0.5 0.5 0.5 1.0]  GraphicAmbientColor=[0.15 0.15 0.15 1.0]  GraphicEmissiveColor=[0.0 0.0 0.0 1.0]  GraphicShininess=75  DoExposeReferenceFrame=on  SerializedFrames=<Frames/>
  HP : PMIOPort  Side=Right
  Spr : PMIOPort  Port=2  Side=Left
  Upr : PMIOPort  Port=3  Side=Left
  ARB : PMIOPort  Port=4  Side=Left
  connections:
  Vis Rack Rod/RConn1 -- Arm/LConn1 -- HP/RConn1 -- Transform Arm Center/LConn1
  Upr/RConn1 -- Arm/RConn1 -- Vis Upright Steer/RConn1
  Arm ARB/RConn1 -- ARB/RConn1
  Transform Arm Center/RConn1 -- Arm Spring/LConn1 -- Arm ARB/LConn1
  Spr/RConn1 -- Arm Spring/RConn1

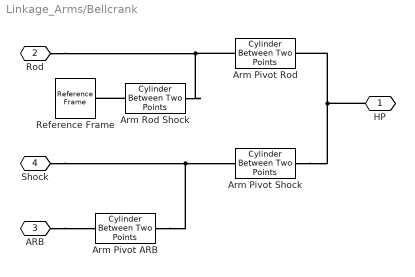
== system Linkage_Arms/Bellcrank ==
  Arm Pivot ARB : Suspension_Utilities/Cylinder Between Two Points  hp_b=hp_bcr_shock.*rhs_hp  hp_f=hp_arb.*rhs_hp  Mass=bcr_mass*0.001  clr_solid=clr_bcr  opc_solid=opc_bcr  rad_solid=radius_bcr
  Arm Pivot Rod : Suspension_Utilities/Cylinder Between Two Points  hp_b=hp_bcr_pivot.*rhs_hp  hp_f=hp_rod.*rhs_hp  Mass=bcr_mass/3  clr_solid=clr_bcr  opc_solid=opc_bcr  rad_solid=radius_bcr
  Arm Pivot Shock : Suspension_Utilities/Cylinder Between Two Points  hp_b=hp_bcr_pivot.*rhs_hp  hp_f=hp_bcr_shock.*rhs_hp  Mass=bcr_mass/3  clr_solid=clr_bcr  opc_solid=opc_bcr  rad_solid=radius_bcr
  Arm Rod Shock : Suspension_Utilities/Cylinder Between Two Points  hp_b=hp_rod.*rhs_hp  hp_f=hp_bcr_shock.*rhs_hp  Mass=bcr_mass/3  clr_solid=clr_bcr  opc_solid=opc_bcr  rad_solid=radius_bcr
  Reference Frame : sm_lib/Frames and Transforms/Reference Frame
  HP : PMIOPort  Side=Right
  Rod : PMIOPort  Port=2  Side=Left
  ARB : PMIOPort  Port=3  Side=Left
  Shock : PMIOPort  Port=4  Side=Left
  connections:
  Arm Rod Shock/RConn1 -- Reference Frame/RConn1
  Shock/RConn1 -- Arm Pivot ARB/LConn1 -- Arm Pivot Shock/RConn1
  HP/RConn1 -- Arm Pivot Rod/LConn1 -- Arm Pivot Shock/LConn1
  Rod/RConn1 -- Arm Pivot Rod/RConn1 -- Arm Rod Shock/LConn1
  ARB/RConn1 -- Arm Pivot ARB/RConn1

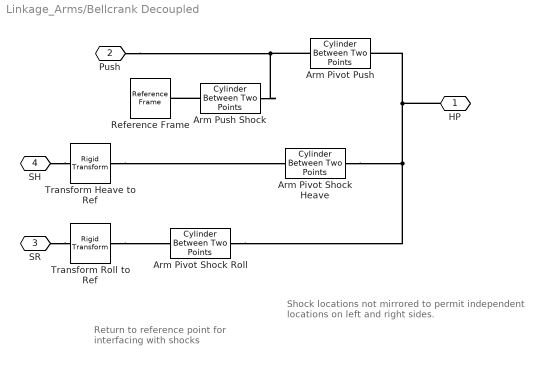
== system Linkage_Arms/Bellcrank Decoupled ==
  note: Return to reference point for interfacing with shocks
  note: Shock locations not mirrored to permit independent locations on left and right sides.
  Arm Pivot Push : Suspension_Utilities/Cylinder Between Two Points  hp_b=hp_bcr_pivot.*rhs_hp  hp_f=hp_pushrod.*rhs_hp  Mass=bcr_mass/3  clr_solid=clr_bcr  opc_solid=opc_bcr  rad_solid=radius_bcr
  Arm Pivot Shock Heave : Suspension_Utilities/Cylinder Between Two Points  hp_b=hp_bcr_pivot.*rhs_hp  hp_f=hp_bcr_shock_heave  Mass=bcr_mass/3  clr_solid=clr_bcr  opc_solid=opc_bcr  rad_solid=radius_bcr
  Arm Pivot Shock Roll : Suspension_Utilities/Cylinder Between Two Points  hp_b=hp_bcr_pivot.*rhs_hp  hp_f=hp_bcr_shock_roll  Mass=bcr_mass*0.001  clr_solid=clr_bcr  opc_solid=opc_bcr  rad_solid=radius_bcr
  Arm Push Shock : Suspension_Utilities/Cylinder Between Two Points  hp_b=hp_pushrod.*rhs_hp  hp_f=hp_bcr_shock_heave  Mass=bcr_mass/3  clr_solid=clr_bcr  opc_solid=opc_bcr  rad_solid=radius_bcr
  Reference Frame : sm_lib/Frames and Transforms/Reference Frame
  Transform Heave to Ref : sm_lib/Frames and Transforms/Rigid Transform  RotationMethod=None  FollAlignAxisA=+X  BaseAlignAxisA=+Y  FollAlignAxisB=+Y  BaseAlignAxisB=+Z  RotationStandardAxis=+Z  RotationAngle=0.0  RotationAngleUnits=deg  RotationArbitraryAxis=[0 0 1]  RotationSequenceAxes=FollowerAxes  RotationSequence=XYX  RotationSequenceAngles=[0 0 0]  RotationSequenceAnglesUnits=deg  RotationMatrix=[1 0 0; 0 1 0; 0 0 1]  Quaternion=[1 0 0 0]  TranslationMethod=Cartesian  TranslationCartesianOffset=hp_bcr_shock_heave  TranslationCartesianOffsetUnits=m  TranslationStandardAxis=+Z  TranslationStandardOffset=0  TranslationStandardOffsetUnits=m  TranslationROffset=0  TranslationROffsetUnits=m  TranslationThetaOffset=0  TranslationThetaOffsetUnits=deg  TranslationZOffset=0  TranslationZOffsetUnits=m
  Transform Roll to Ref : sm_lib/Frames and Transforms/Rigid Transform  RotationMethod=None  FollAlignAxisA=+X  BaseAlignAxisA=+Y  FollAlignAxisB=+Y  BaseAlignAxisB=+Z  RotationStandardAxis=+Z  RotationAngle=0.0  RotationAngleUnits=deg  RotationArbitraryAxis=[0 0 1]  RotationSequenceAxes=FollowerAxes  RotationSequence=XYX  RotationSequenceAngles=[0 0 0]  RotationSequenceAnglesUnits=deg  RotationMatrix=[1 0 0; 0 1 0; 0 0 1]  Quaternion=[1 0 0 0]  TranslationMethod=Cartesian  TranslationCartesianOffset=hp_bcr_shock_roll  TranslationCartesianOffsetUnits=m  TranslationStandardAxis=+Z  TranslationStandardOffset=0  TranslationStandardOffsetUnits=m  TranslationROffset=0  TranslationROffsetUnits=m  TranslationThetaOffset=0  TranslationThetaOffsetUnits=deg  TranslationZOffset=0  TranslationZOffsetUnits=m
  HP : PMIOPort  Side=Right
  Push : PMIOPort  Port=2  Side=Left
  SR : PMIOPort  Port=3  Side=Left
  SH : PMIOPort  Port=4  Side=Left
  connections:
  SR/RConn1 -- Transform Roll to Ref/LConn1
  Arm Push Shock/LConn1 -- Arm Pivot Push/RConn1 -- Push/RConn1
  Arm Pivot Shock Heave/LConn1 -- Arm Pivot Shock Roll/LConn1 -- Arm Pivot Push/LConn1 -- HP/RConn1
  SH/RConn1 -- Transform Heave to Ref/LConn1
  Arm Push Shock/RConn1 -- Reference Frame/RConn1
  Transform Roll to Ref/RConn1 -- Arm Pivot Shock Roll/RConn1
  Transform Heave to Ref/RConn1 -- Arm Pivot Shock Heave/RConn1

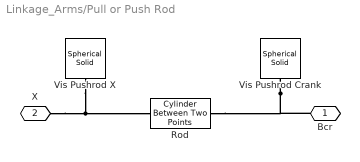
== system Linkage_Arms/Pull or Push Rod ==
  Rod : Suspension_Utilities/Cylinder Between Two Points  hp_b=hp_in.*[1 rhs_rod 1]  hp_f=hp_out.*[1 rhs_rod 1]  Mass=rod_mass  clr_solid=clr_rod  opc_solid=opc_rod  rad_solid=radius_rod
  Vis Pushrod Crank : sm_lib/Body Elements/Spherical Solid  SphereRadius=size_conn_rod  SphereRadiusUnits=m  ExportEntireGeometry=off  InertiaType=CalculateFromGeometry  BasedOnType=Density  Density=0  DensityUnits=kg/m^3  Mass=1  MassUnits=kg  CenterOfMass=[0 0 0]  CenterOfMassUnits=m  MomentsOfInertia=[1 1 1]  MomentsOfInertiaUnits=kg*m^2  ProductsOfInertia=[0 0 0]  ProductsOfInertiaUnits=kg*m^2  GraphicType=FromGeometry  MarkerShape=Sphere  MarkerSize=10  GraphicVisPropType=SimpleVisualProperties  GraphicDiffuseColor=clr_conn_rod  GraphicOpacity=opc_conn_rod  GraphicSpecularColor=[0.5 0.5 0.5 1.0]  GraphicAmbientColor=[0.15 0.15 0.15 1.0]  GraphicEmissiveColor=[0.0 0.0 0.0 1.0]  GraphicShininess=75  DoExposeReferenceFrame=on  SerializedFrames=<Frames/>
  Vis Pushrod X : sm_lib/Body Elements/Spherical Solid  SphereRadius=size_conn_rod  SphereRadiusUnits=m  ExportEntireGeometry=off  InertiaType=CalculateFromGeometry  BasedOnType=Density  Density=0  DensityUnits=kg/m^3  Mass=1  MassUnits=kg  CenterOfMass=[0 0 0]  CenterOfMassUnits=m  MomentsOfInertia=[1 1 1]  MomentsOfInertiaUnits=kg*m^2  ProductsOfInertia=[0 0 0]  ProductsOfInertiaUnits=kg*m^2  GraphicType=FromGeometry  MarkerShape=Sphere  MarkerSize=10  GraphicVisPropType=SimpleVisualProperties  GraphicDiffuseColor=clr_conn_rod  GraphicOpacity=opc_conn_rod  GraphicSpecularColor=[0.5 0.5 0.5 1.0]  GraphicAmbientColor=[0.15 0.15 0.15 1.0]  GraphicEmissiveColor=[0.0 0.0 0.0 1.0]  GraphicShininess=75  DoExposeReferenceFrame=on  SerializedFrames=<Frames/>
  Bcr : PMIOPort  Side=Right
  X : PMIOPort  Port=2  Side=Left
  connections:
  Vis Pushrod Crank/RConn1 -- Bcr/RConn1 -- Rod/LConn1
  X/RConn1 -- Rod/RConn1 -- Vis Pushrod X/RConn1
